simulink model "Aufgabe9"  (R2016a)
settings: Solver=VariableStepAuto  StartTime=0.0  StopTime=1.5  RelTol=1e-3
libraries: simulink x2
settings Model: Creator=Bornitz  LastModifiedBy=Bornitz

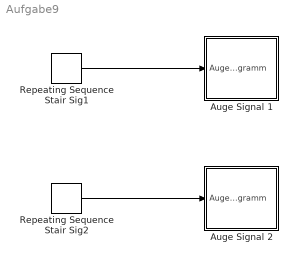
== system Aufgabe9 ==
  Auge Signal 1 : Subsystem
  Auge Signal 2 : Subsystem
  Repeating Sequence Stair Sig1 : simulink/Sources/Repeating Sequence Stair  OutValues=sig1  tsamp=1/(16*5000)  OutMin=[]  OutMax=[]  OutDataTypeStr=double  OutputDataTypeScalingMode=double  OutDataType=fixdt(0,8)  ConRadixGroup=Best Precision: Vector-wise  OutScaling=2^-12
  Repeating Sequence Stair Sig2 : simulink/Sources/Repeating Sequence Stair  OutValues=sig2  tsamp=1/(16*5000)  OutMin=[]  OutMax=[]  OutDataTypeStr=double  OutputDataTypeScalingMode=double  OutDataType=fixdt(0,8)  ConRadixGroup=Best Precision: Vector-wise  OutScaling=2^-12
  wires:
  Repeating Sequence Stair Sig1/1 -> Auge Signal 1/1(Augendiagramm)
  Repeating Sequence Stair Sig2/1 -> Auge Signal 2/1(Augendiagramm)

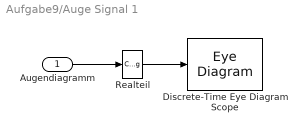
== system Aufgabe9/Auge Signal 1 ==
  Augendiagramm : Inport
  Discrete-Time Eye Diagram Scope : EyeDiagram  Tag=EyeDiagram
  Realteil : ComplexToRealImag  Output=Real
  wires:
  Realteil/1 -> Discrete-Time Eye Diagram Scope/1
  Augendiagramm/1 -> Realteil/1

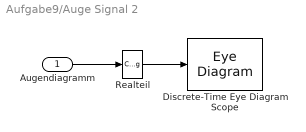
== system Aufgabe9/Auge Signal 2 ==
  Augendiagramm : Inport
  Discrete-Time Eye Diagram Scope : EyeDiagram  Tag=EyeDiagram
  Realteil : ComplexToRealImag  Output=Real
  wires:
  Realteil/1 -> Discrete-Time Eye Diagram Scope/1
  Augendiagramm/1 -> Realteil/1
